simulink model "WF_onshore"  (R2024a)
settings: Solver=VariableStepAuto  StartTime=0  StopTime=0.9  RelTol=1e-3
values from neighbouring files (symbols this model uses):
  WF = calculate_WF(WF)    [WF_parameter_variation.m]
undefined symbols (not defined in the file or in its folder): L, Lg, R
libraries: spsSeriesRLCBranchLib x15, simulink_extras x8, spsThreePhaseVIMeasurementLib x6, spsControlledVoltageSourceLib x6, simulink x4, spsGroundLib x3, spsVariableInductorLib x3, spsThreePhaseTransformerTwoWindingsLib x2, powerlib_extras x1, spspowerguiLib x1
(part 2 of 2)

== system WF_onshore/WT_aggregated/Transformations (pu and dq)/Park ==
  x_abc : Inport
  delta : Inport  Port=2
  Demux1 : Demux  Outputs=3
  Fcn : Fcn  Expr=2/3*(cos(u(4))*u(1)+cos(u(4)-2/3*pi)*u(2)+cos(u(4)+2/3*pi)*u(3))
  Fcn1 : Fcn  Expr=-2/3*(sin(u(4))*u(1)+sin(u(4)-2/3*pi)*u(2)+sin(u(4)+2/3*pi)*u(3))
  Mux : Mux
  Mux1 : Mux  Inputs=2
  x_dq : Outport
  wires:
  Demux1/1 -> Mux/1
  Demux1/2 -> Mux/2
  Demux1/3 -> Mux/3
  x_abc/1 -> Demux1/1
  delta/1 -> Mux/4
  Mux/1 -> Fcn/1, Fcn1/1
  Fcn/1 -> Mux1/1
  Fcn1/1 -> Mux1/2
  Mux1/1 -> x_dq/1

== system WF_onshore/WT_aggregated/Transformations (pu and dq)/Park1 ==
  x_abc : Inport
  delta : Inport  Port=2
  Demux1 : Demux  Outputs=3
  Fcn : Fcn  Expr=2/3*(cos(u(4))*u(1)+cos(u(4)-2/3*pi)*u(2)+cos(u(4)+2/3*pi)*u(3))
  Fcn1 : Fcn  Expr=-2/3*(sin(u(4))*u(1)+sin(u(4)-2/3*pi)*u(2)+sin(u(4)+2/3*pi)*u(3))
  Mux : Mux
  Mux1 : Mux  Inputs=2
  x_dq : Outport
  wires:
  Mux1/1 -> x_dq/1
  Fcn1/1 -> Mux1/2
  Fcn/1 -> Mux1/1
  Mux/1 -> Fcn1/1, Fcn/1
  delta/1 -> Mux/4
  x_abc/1 -> Demux1/1
  Demux1/3 -> Mux/3
  Demux1/2 -> Mux/2
  Demux1/1 -> Mux/1

== system WF_onshore/WT_aggregated/Transformations (pu and dq)/Park2 ==
  x_abc : Inport
  delta : Inport  Port=2
  Demux1 : Demux  Outputs=3
  Fcn : Fcn  Expr=2/3*(cos(u(4))*u(1)+cos(u(4)-2/3*pi)*u(2)+cos(u(4)+2/3*pi)*u(3))
  Fcn1 : Fcn  Expr=-2/3*(sin(u(4))*u(1)+sin(u(4)-2/3*pi)*u(2)+sin(u(4)+2/3*pi)*u(3))
  Mux : Mux
  Mux1 : Mux  Inputs=2
  x_dq : Outport
  wires:
  Mux1/1 -> x_dq/1
  Fcn1/1 -> Mux1/2
  Fcn/1 -> Mux1/1
  Mux/1 -> Fcn1/1, Fcn/1
  delta/1 -> Mux/4
  x_abc/1 -> Demux1/1
  Demux1/3 -> Mux/3
  Demux1/2 -> Mux/2
  Demux1/1 -> Mux/1

== system WF_onshore/WT_aggregated/Transformations (pu and dq)/Park4 ==
  x_abc : Inport
  delta : Inport  Port=2
  Demux1 : Demux  Outputs=3
  Fcn : Fcn  Expr=2/3*(cos(u(4))*u(1)+cos(u(4)-2/3*pi)*u(2)+cos(u(4)+2/3*pi)*u(3))
  Fcn1 : Fcn  Expr=-2/3*(sin(u(4))*u(1)+sin(u(4)-2/3*pi)*u(2)+sin(u(4)+2/3*pi)*u(3))
  Mux : Mux
  Mux1 : Mux  Inputs=2
  x_dq : Outport
  wires:
  Mux1/1 -> x_dq/1
  Fcn1/1 -> Mux1/2
  Fcn/1 -> Mux1/1
  Mux/1 -> Fcn1/1, Fcn/1
  delta/1 -> Mux/4
  x_abc/1 -> Demux1/1
  Demux1/3 -> Mux/3
  Demux1/2 -> Mux/2
  Demux1/1 -> Mux/1

== system WF_onshore/WT_aggregated/Transformations (pu and dq)/Subsystem2 ==
  x_dq : Inport
  Demux : Demux  Outputs=2
  Real-Imag to Complex : RealImagToComplex
  x_d+ix_q : Outport
  wires:
  Demux/1 -> Real-Imag to Complex/1
  Demux/2 -> Real-Imag to Complex/2
  x_dq/1 -> Demux/1
  Real-Imag to Complex/1 -> x_d+ix_q/1

== system WF_onshore/WT_aggregated/Transformations (pu and dq)/Subsystem3 ==
  x_dq : Inport
  Demux : Demux  Outputs=2
  Real-Imag to Complex : RealImagToComplex
  x_d+ix_q : Outport
  wires:
  Demux/1 -> Real-Imag to Complex/1
  Demux/2 -> Real-Imag to Complex/2
  x_dq/1 -> Demux/1
  Real-Imag to Complex/1 -> x_d+ix_q/1

== system WF_onshore/WT_aggregated/Transformations (pu and dq)/Subsystem4 ==
  x_dq : Inport
  Demux : Demux  Outputs=2
  Real-Imag to Complex : RealImagToComplex
  x_d+ix_q : Outport
  wires:
  Demux/1 -> Real-Imag to Complex/1
  Demux/2 -> Real-Imag to Complex/2
  x_dq/1 -> Demux/1
  Real-Imag to Complex/1 -> x_d+ix_q/1

== system WF_onshore/WT_aggregated/Transformations (pu and dq)/Subsystem7 ==
  x_dq : Inport
  Demux : Demux  Outputs=2
  Real-Imag to Complex : RealImagToComplex
  x_d+ix_q : Outport
  wires:
  Real-Imag to Complex/1 -> x_d+ix_q/1
  x_dq/1 -> Demux/1
  Demux/2 -> Real-Imag to Complex/2
  Demux/1 -> Real-Imag to Complex/1

== system WF_onshore/WT_aggregated/Control System/Current controller/Subsystem ==
  x : Inport
  x0 : Inport  Port=2
  Complex to Real-Imag : ComplexToRealImag
  Complex to Real-Imag1 : ComplexToRealImag
  Integrator : Integrator  InitialConditionSource=external  AbsoluteTolerance=1e-10
  Integrator1 : Integrator  InitialConditionSource=external  AbsoluteTolerance=1e-15
  Real-Imag to Complex : RealImagToComplex
  x/s : Outport
  wires:
  Complex to Real-Imag/1 -> Integrator/1
  Complex to Real-Imag1/1 -> Integrator/2
  Complex to Real-Imag1/2 -> Integrator1/2
  x/1 -> Complex to Real-Imag/1
  Real-Imag to Complex/1 -> x/s/1
  x0/1 -> Complex to Real-Imag1/1
  Integrator1/1 -> Real-Imag to Complex/2
  Integrator/1 -> Real-Imag to Complex/1
  Complex to Real-Imag/2 -> Integrator1/1

== system WF_onshore/WT_aggregated/Control System/Current controller/Subsystem1 ==
  in : Inport
  Demux : Demux  Outputs=2
  Mux : Mux  Inputs=2
  Subsystem3 : Subsystem
  Subsystem6 : Subsystem
  Transfer Fcn (with initial outputs) : simulink_extras/Additional Linear/Transfer Fcn (with initial outputs)  N=[Omega]  D="[1  Omega]"  Y0=xd0  U0=xd0
  Transfer Fcn (with initial outputs)1 : simulink_extras/Additional Linear/Transfer Fcn (with initial outputs)  N=[Omega]  D="[1  Omega]"  Y0=xq0  U0=xq0
  out : Outport
  wires:
  Transfer Fcn (with initial outputs)/1 -> Mux/1
  Transfer Fcn (with initial outputs)1/1 -> Mux/2
  Mux/1 -> Subsystem3/1(x_dq)
  Subsystem6/1(x_dq) -> Demux/1
  in/1 -> Subsystem6/1(x_d+ix_q)
  Subsystem3/1(x_d+ix_q) -> out/1
  Demux/1 -> Transfer Fcn (with initial outputs)/1
  Demux/2 -> Transfer Fcn (with initial outputs)1/1

== system WF_onshore/WT_aggregated/Control System/GFL state space/Subsystem5 ==
  x_d+ix_q : Inport
  Complex to Real-Imag2 : ComplexToRealImag
  Mux : Mux  Inputs=2
  x_dq : Outport
  wires:
  Complex to Real-Imag2/1 -> Mux/1
  Complex to Real-Imag2/2 -> Mux/2
  Mux/1 -> x_dq/1
  x_d+ix_q/1 -> Complex to Real-Imag2/1

== system WF_onshore/WT_aggregated/Control System/GFL state space/Subsystem8 ==
  x_d+ix_q : Inport
  Complex to Real-Imag2 : ComplexToRealImag
  Mux : Mux  Inputs=2
  x_dq : Outport
  wires:
  Complex to Real-Imag2/1 -> Mux/1
  Complex to Real-Imag2/2 -> Mux/2
  Mux/1 -> x_dq/1
  x_d+ix_q/1 -> Complex to Real-Imag2/1

== system WF_onshore/WT_aggregated/Control System/GFL state space/Subsystem9 ==
  x_d+ix_q : Inport
  Complex to Real-Imag2 : ComplexToRealImag
  Mux : Mux  Inputs=2
  x_dq : Outport
  wires:
  Complex to Real-Imag2/1 -> Mux/1
  Complex to Real-Imag2/2 -> Mux/2
  Mux/1 -> x_dq/1
  x_d+ix_q/1 -> Complex to Real-Imag2/1

== system WF_onshore/WT_aggregated/Control System/GFM State Space model/Subsystem5 ==
  x_d+ix_q : Inport
  Complex to Real-Imag2 : ComplexToRealImag
  Mux : Mux  Inputs=2
  x_dq : Outport
  wires:
  x_d+ix_q/1 -> Complex to Real-Imag2/1
  Mux/1 -> x_dq/1
  Complex to Real-Imag2/2 -> Mux/2
  Complex to Real-Imag2/1 -> Mux/1

== system WF_onshore/WT_aggregated/Control System/GFM State Space model/Subsystem8 ==
  x_d+ix_q : Inport
  Complex to Real-Imag2 : ComplexToRealImag
  Mux : Mux  Inputs=2
  x_dq : Outport
  wires:
  x_d+ix_q/1 -> Complex to Real-Imag2/1
  Mux/1 -> x_dq/1
  Complex to Real-Imag2/2 -> Mux/2
  Complex to Real-Imag2/1 -> Mux/1

== system WF_onshore/WT_aggregated/Control System/GFM State Space model/Subsystem9 ==
  x_d+ix_q : Inport
  Complex to Real-Imag2 : ComplexToRealImag
  Mux : Mux  Inputs=2
  x_dq : Outport
  wires:
  x_d+ix_q/1 -> Complex to Real-Imag2/1
  Mux/1 -> x_dq/1
  Complex to Real-Imag2/2 -> Mux/2
  Complex to Real-Imag2/1 -> Mux/1

== system WF_onshore/WT_aggregated/Control System/PLL1/Subsystem1 ==
  x_d+ix_q : Inport
  Complex to Real-Imag2 : ComplexToRealImag
  Mux : Mux  Inputs=2
  x_dq : Outport
  wires:
  x_d+ix_q/1 -> Complex to Real-Imag2/1
  Mux/1 -> x_dq/1
  Complex to Real-Imag2/2 -> Mux/2
  Complex to Real-Imag2/1 -> Mux/1

== system WF_onshore/WT_aggregated/Control System/PLL1/Subsystem3 ==
  x_dq : Inport
  Demux : Demux  Outputs=2
  Real-Imag to Complex : RealImagToComplex
  x_d+ix_q : Outport
  wires:
  Demux/1 -> Real-Imag to Complex/1
  Demux/2 -> Real-Imag to Complex/2
  x_dq/1 -> Demux/1
  Real-Imag to Complex/1 -> x_d+ix_q/1

== system WF_onshore/WT_aggregated/Control System/PQ controller/Subsystem3 ==
  x_dq : Inport
  Demux : Demux  Outputs=2
  Real-Imag to Complex : RealImagToComplex
  x_d+ix_q : Outport
  wires:
  Demux/1 -> Real-Imag to Complex/1
  Demux/2 -> Real-Imag to Complex/2
  x_dq/1 -> Demux/1
  Real-Imag to Complex/1 -> x_d+ix_q/1

== system WF_onshore/WT_aggregated/Control System/Voltage controller DEM/Subsystem ==
  x : Inport
  x0 : Inport  Port=2
  Complex to Real-Imag : ComplexToRealImag
  Complex to Real-Imag1 : ComplexToRealImag
  Integrator : Integrator  InitialConditionSource=external
  Integrator1 : Integrator  InitialConditionSource=external
  Real-Imag to Complex : RealImagToComplex
  x/s : Outport
  wires:
  Complex to Real-Imag/1 -> Integrator1/1
  Complex to Real-Imag/2 -> Integrator/1
  Complex to Real-Imag1/1 -> Integrator1/2
  Complex to Real-Imag1/2 -> Integrator/2
  x/1 -> Complex to Real-Imag/1
  Real-Imag to Complex/1 -> x/s/1
  x0/1 -> Complex to Real-Imag1/1
  Integrator1/1 -> Real-Imag to Complex/1
  Integrator/1 -> Real-Imag to Complex/2

== system WF_onshore/WT_aggregated/Control System/Voltage controller QSEM/Subsystem2 ==
  x_d+ix_q : Inport
  Complex to Real-Imag2 : ComplexToRealImag
  Mux : Mux  Inputs=2
  x_dq : Outport
  wires:
  x_d+ix_q/1 -> Complex to Real-Imag2/1
  Mux/1 -> x_dq/1
  Complex to Real-Imag2/2 -> Mux/2
  Complex to Real-Imag2/1 -> Mux/1

== system WF_onshore/WT_aggregated/Control System/Voltage controller QSEM/Subsystem3 ==
  x_dq : Inport
  Demux : Demux  Outputs=2
  Real-Imag to Complex : RealImagToComplex
  x_d+ix_q : Outport
  wires:
  Demux/1 -> Real-Imag to Complex/1
  Demux/2 -> Real-Imag to Complex/2
  x_dq/1 -> Demux/1
  Real-Imag to Complex/1 -> x_d+ix_q/1

== system WF_onshore/WT_aggregated/Control System/Voltage controller VCVSM/Subsystem ==
  x : Inport
  x0 : Inport  Port=2
  Complex to Real-Imag : ComplexToRealImag
  Complex to Real-Imag1 : ComplexToRealImag
  Integrator : Integrator  InitialConditionSource=external
  Integrator1 : Integrator  InitialConditionSource=external
  Real-Imag to Complex : RealImagToComplex
  x/s : Outport
  wires:
  Complex to Real-Imag/1 -> Integrator1/1
  Complex to Real-Imag/2 -> Integrator/1
  Complex to Real-Imag1/1 -> Integrator1/2
  Complex to Real-Imag1/2 -> Integrator/2
  x/1 -> Complex to Real-Imag/1
  Real-Imag to Complex/1 -> x/s/1
  x0/1 -> Complex to Real-Imag1/1
  Integrator1/1 -> Real-Imag to Complex/1
  Integrator/1 -> Real-Imag to Complex/2

== system WF_onshore/WT_aggregated/Control System/Current controller/Subsystem1/Subsystem3 ==
  x_dq : Inport
  Demux : Demux  Outputs=2
  Real-Imag to Complex : RealImagToComplex
  x_d+ix_q : Outport
  wires:
  Demux/1 -> Real-Imag to Complex/1
  Demux/2 -> Real-Imag to Complex/2
  x_dq/1 -> Demux/1
  Real-Imag to Complex/1 -> x_d+ix_q/1

== system WF_onshore/WT_aggregated/Control System/Current controller/Subsystem1/Subsystem6 ==
  x_d+ix_q : Inport
  Complex to Real-Imag2 : ComplexToRealImag
  Mux : Mux  Inputs=2
  x_dq : Outport
  wires:
  Complex to Real-Imag2/1 -> Mux/1
  Complex to Real-Imag2/2 -> Mux/2
  Mux/1 -> x_dq/1
  x_d+ix_q/1 -> Complex to Real-Imag2/1
